simulink model "clgproject"  (Simulink 7.5)
settings: Solver=ode45  StartTime=0.0  StopTime=10.0  RelTol=1e-3
undefined symbols (not defined in the file): Hydride, Metal, Nickel
libraries: powerlib x9, dspstat3 x2, electricdrivelib x1, elec_lib x1, powerlib_extras x1, simulink x1
settings Model: Creator=NAGASAI PRAKASH  LastModifiedBy=NAGASAI PRAKASH

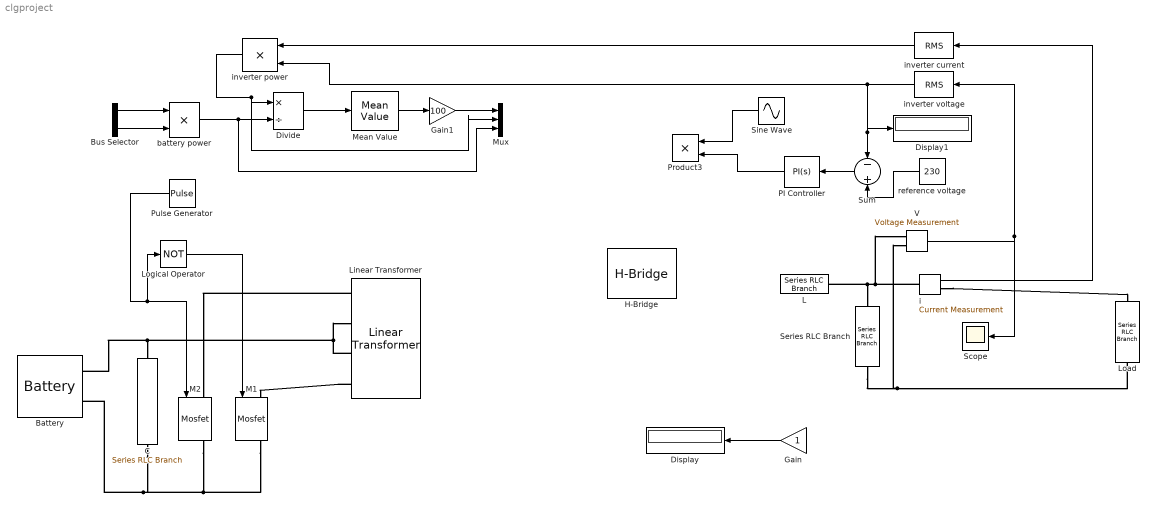
== system clgproject ==
  Battery : electricdrivelib/Extra Sources/Battery  DialogController=POWERSYS.PowerSysDialog  SystemSampleTime=-1  BatType=Nickel-Metal-Hydride  ShowDetailedParameters=off  NomV=1.2  NomQ=1.5  SOC=100  PresetModel=on  MaxQ=1.6154  FullV=1.4136  Dis_rate=0.3  R=0.008  Normal_OP=1.4423  expZone="[1.3017         0.3]"  Dis_Char=off  current=[1.5 3]  Units=Ampere-hour  Batt_Tr=30
  Bus Selector : BusSelector  OutputSignals=signal1,signal2
  C : powerlib/Elements/Series RLC Branch  DialogController=POWERSYS.PowerSysDialog  PhysicalDomain=powersysdomain  SubClassName=unknown  LeftPortType=p1  RightPortType=p1  LConnTagsString=__new0  RConnTagsString=__new0  BranchType=C  Resistance=1  Inductance=1e-3  SetiL0=off  InitialCurrent=0  Capacitance=1e-6  Setx0=off  InitialVoltage=0  Measurements=None
  Display : Display
      settings: Decimation=3
  Display1 : Display
      settings: Decimation=3
  Divide : Product  Inputs=*/  OutDataType=fixdt(1, 16)  OutScaling=2^-10
  Gain : Gain  ParameterDataType=fixdt(1, 16)  ParameterScaling=2^0  OutDataType=fixdt(1, 16)  OutScaling=2^0
  Gain1 : Gain  Gain=100  ParameterDataType=fixdt(1, 16)  ParameterScaling=2^0  OutDataType=fixdt(1, 16)  OutScaling=2^0
  H-Bridge : elec_lib/Actuators & Drivers/Drivers/H-Bridge  DialogController=NetworkEngine.DynNeDlgSource  SystemSampleTime=-1  Venable=2.5 V  Vmax=5 V  Vreverse=2.5 V  Vbrake=2.5 V  Vm=12 V  pwm_or_av=1  freewheeling_mode=1  Ron=0.1 Ohm  Don=0.05 Ohm  current_Log=off  voltage_Log=off  power_Log=off  LocalVarNames=|current|voltage|power  LocalVarDescs=|Load current (A)|Load voltage (V)|Load power (W)  LocalVarLogging=[0 0 0]
  L : powerlib/Elements/Series RLC Branch  DialogController=POWERSYS.PowerSysDialog  PhysicalDomain=powersysdomain  SubClassName=unknown  LeftPortType=p1  RightPortType=p1  LConnTagsString=__new0  RConnTagsString=__new0  BranchType=L  Resistance=1  Inductance=1e-3  SetiL0=off  InitialCurrent=0  Capacitance=1e-6  Setx0=off  InitialVoltage=0  Measurements=None
  Linear Transformer : powerlib/Elements/Linear Transformer  DialogController=POWERSYS.PowerSysDialog  PhysicalDomain=powersysdomain  SubClassName=unknown  LeftPortType=p1  RightPortType=p1  LConnTagsString=a|b  RConnTagsString=A|B|C|D  UNITS=pu  NominalPower=[ 250e6 60 ]  winding1="[ 735e3  0.002  0.08 ]"  winding2="[ 315e3  0.002  0.08 ]"  ThreeWindings=on  winding3=[ 315e3 0.002 0.08 ]  RmLm=[ 500 500 ]  Measurements=None  DataType=off
  Load : powerlib/Elements/Series RLC Branch  DialogController=POWERSYS.PowerSysDialog  PhysicalDomain=powersysdomain  SubClassName=unknown  LeftPortType=p1  RightPortType=p1  LConnTagsString=__new0  RConnTagsString=__new0  BranchType=R  Resistance=1  Inductance=1e-3  SetiL0=off  InitialCurrent=0  Capacitance=1e-6  Setx0=off  InitialVoltage=0  Measurements=None
  Logical Operator : Logic  Operator=NOT  AllPortsSameDT=off  OutDataTypeMode=boolean  LogicDataType=fixdt(0, 8)  OutDataTypeStr=boolean
  M1 : powerlib/Power Electronics/Mosfet  DialogController=POWERSYS.PowerSysDialog  SystemSampleTime=-1  Ron=0.1  Lon=0  Rd=0.01  Vfd=0  IC=0  Rs=1e5  Cs=inf  Measurements=on
  M2 : powerlib/Power Electronics/Mosfet  DialogController=POWERSYS.PowerSysDialog  SystemSampleTime=-1  Ron=0.1  Lon=0  Rd=0.01  Vfd=0  IC=0  Rs=1e5  Cs=inf  Measurements=on
  Mean Value : powerlib_extras/Measurements/Mean Value  DialogController=POWERSYS.PowerSysDialog  SystemSampleTime=-1  Period=1/60
  Mux : Mux  Inputs=3
  PI Controller : simulink/Continuous/PID Controller  DialogController=pidpack.PIDConfig.pidDDGCreate  DialogControllerArgs=DataTag0  SystemSampleTime=-1  Controller=PI  TimeDomain=Continuous-time  SampleTime=1  IntegratorMethod=Forward Euler  FilterMethod=Forward Euler  Form=Parallel  P=1  I=1  D=0  N=100  InitialConditionSource=internal  InitialConditionForIntegrator=0  InitialConditionForFilter=0  ExternalReset=none  LimitOutput=off  UpperSaturationLimit=inf  LowerSaturationLimit=-inf  LinearizeAsGain=off  AntiWindupMode=none  Kb=1  TrackingMode=off  Kt=1  PParamMin=[]  PParamMax=[]  IParamMin=[]  IParamMax=[]  DParamMin=[]  DParamMax=[]  NParamMin=[]  NParamMax=[]  KbParamMin=[]  KbParamMax=[]  KtParamMin=[]  KtParamMax=[]  POutMin=[]  POutMax=[]  IOutMin=[]  IOutMax=[]  DOutMin=[]  DOutMax=[]  NOutMin=[]  NOutMax=[]  KbOutMin=[]  KbOutMax=[]  KtOutMin=[]  KtOutMax=[]  IntegratorOutMin=[]  IntegratorOutMax=[]  FilterOutMin=[]  FilterOutMax=[]  SumOutMin=[]  SumOutMax=[]  SumI1OutMin=[]  SumI1OutMax=[]  SumI2OutMin=[]  SumI2OutMax=[]  SumI3OutMin=[]  SumI3OutMax=[]  SumDOutMin=[]  SumDOutMax=[]  SaturationOutMin=[]  SaturationOutMax=[]  IntegratorContinuousStateAttributes=''  IntegratorStateMustResolveToSignalObject=off  IntegratorRTWStateStorageClass=Auto  FilterContinuousStateAttributes=''  FilterStateMustResolveToSignalObject=off  FilterRTWStateStorageClass=Auto
  Product3 : Product  OutDataType=fixdt(1, 16)  OutScaling=2^0  RndMeth=Zero
  Pulse Generator : DiscretePulseGenerator  PulseType=Time based  Amplitude=1  Period=10  PulseWidth=5  PhaseDelay=0  SampleTime=1
  Scope : Scope
  Series RLC Branch : powerlib/Elements/Series RLC Branch  DialogController=POWERSYS.PowerSysDialog  PhysicalDomain=powersysdomain  SubClassName=unknown  LeftPortType=p1  RightPortType=p1  LConnTagsString=__new0  RConnTagsString=__new0  BranchType=C  Resistance=1  Inductance=1e-3  SetiL0=off  InitialCurrent=0  Capacitance=1e-6  Setx0=off  InitialVoltage=0  Measurements=None
  Sine Wave : Sin  Amplitude=1  Bias=0  Frequency=1  Phase=0  Samples=10  SampleTime=0  Offset=0
  Sum : Sum  Inputs=-+  OutDataType=fixdt(1, 16)  OutScaling=2^0
  V : powerlib/Measurements/Voltage Measurement  DialogController=POWERSYS.PowerSysDialog  SystemSampleTime=-1  PhasorSimulation=off  OutputType=Complex  PSBequivalent=0
  battery power : Product  OutDataType=fixdt(1, 16)  OutScaling=2^0  RndMeth=Zero
  i : powerlib/Measurements/Current Measurement  DialogController=POWERSYS.PowerSysDialog  SystemSampleTime=-1  PhasorSimulation=off  OutputType=Complex  PSBequivalent=0
  inverter current : dspstat3/RMS  DialogController=dspDDGCreate  DialogControllerArgs=DataTag1  run=off  reset_popup=None  directionMode=Each column  dimension=1  treatSBRowAsCol=on
  inverter power : Product  OutDataType=fixdt(1, 16)  OutScaling=2^0  RndMeth=Zero
  inverter voltage : dspstat3/RMS  DialogController=dspDDGCreate  DialogControllerArgs=DataTag2  run=off  reset_popup=None  directionMode=Each column  dimension=1  treatSBRowAsCol=on
  reference voltage : Constant  Value=230  OutDataType=fixdt(1, 16)  OutScaling=2^0
  wires:
  Pulse Generator/1 -> M2/1, Logical Operator/1
  Gain/1 -> Display/1
  V/1 -> inverter voltage/1, Scope/1
  i/1 -> inverter current/1
  inverter current/1 -> inverter power/1
  inverter voltage/1 -> inverter power/2, Display1/1, Sum/1
  reference voltage/1 -> Sum/2
  Logical Operator/1 -> M1/1
  Sum/1 -> PI Controller/1
  PI Controller/1 -> Product3/2
  Sine Wave/1 -> Product3/1
  Bus Selector/1 -> battery power/1
  Bus Selector/2 -> battery power/2
  inverter power/1 -> Divide/1, Mux/2
  battery power/1 -> Divide/2, Mux/3
  Divide/1 -> Mean Value/1
  Mean Value/1 -> Gain1/1
  Gain1/1 -> Mux/1
  connections:
  Linear Transformer/RConn3 -- Linear Transformer/RConn2 -- Battery/LConn1 -- C/LConn1
  Linear Transformer/RConn4 -- M1/LConn1
  Linear Transformer/RConn1 -- M2/LConn1
  M1/RConn1 -- M2/RConn1 -- Battery/LConn2 -- C/RConn1
  Series RLC Branch/RConn1 -- Load/LConn1 -- V/LConn2
  i/LConn1 -- L/RConn1 -- Series RLC Branch/LConn1 -- V/LConn1
  i/RConn1 -- Load/RConn1
